simulink model "fuzzyLCSv2"  (R2021b)
settings: Solver=VariableStepAuto  StartTime=0.0  StopTime=inf  RelTol=1e-3
libraries: robotlib x3, fuzblock x1
settings Model: SimulationMode=accelerator  Creator=lucas  LastModifiedBy=lucas

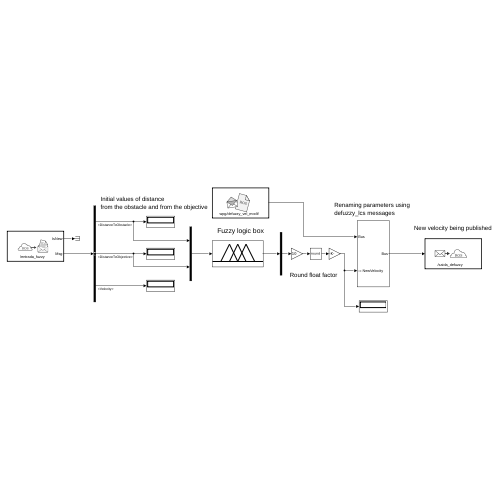
[thumbnail: Simulink's stored preview of the top-level diagram]
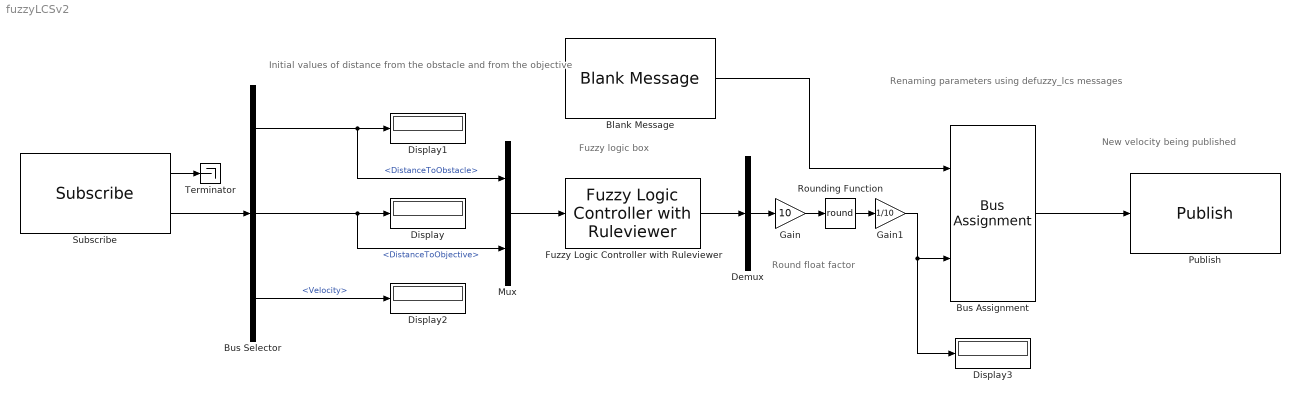
== system fuzzyLCSv2 ==
  note: Renaming parameters using
      | defuzzy_lcs messages
  note: Initial values of distance
      | from the obstacle and from the objective
  note: Fuzzy logic box
  note: New velocity being published
  note: Round float factor
  Blank Message : robotlib/Blank Message  messageClass=Message  entityType=wpg/defuzzy_vel_modif  messageType=wpg/defuzzy_vel_modif  SampleTime=inf  legacyBusStruct=off
  Bus Assignment : BusAssignment  AssignedSignals=NewVelocity
  Bus Selector : BusSelector  OutputSignals=DistanceToObstacle,DistanceToObjective,Velocity
  Demux : Demux  Outputs=1
  Display{,1..3} (4 alike) : Display
      settings: Decimation=2
  Fuzzy Logic Controller with Ruleviewer : fuzblock/Fuzzy Logic  Controller  with Ruleviewer  fismatrix=lucasdist  Ts=2
  Gain : Gain  Gain=10
  Gain1 : Gain  Gain=1/10
  Mux : Mux  Inputs=2
  Publish : robotlib/Publish  topicSource=Specify your own  topic=/saida_defuzzy  messageType=wpg/defuzzy_vel_modif  legacyBusStruct=off  messageQueueLength=1
  Rounding Function : Rounding  Operator=round
  Subscribe : robotlib/Subscribe  topicSource=Specify your own  topic=/entrada_fuzzy  messageType=wpg/fuzzy_vel_modif  SampleTime=-1  legacyBusStruct=off  messageQueueLength=1
  Terminator : Terminator
  wires:
  Subscribe/2 -> Bus Selector/1
  Subscribe/1 -> Terminator/1
  Bus Selector/1 -> Display1/1, Mux/1  "<DistanceToObstacle>"
  Bus Selector/2 -> Display/1, Mux/2  "<DistanceToObjective>"
  Bus Selector/3 -> Display2/1  "<Velocity>"
  Blank Message/1 -> Bus Assignment/1
  Bus Assignment/1 -> Publish/1
  Mux/1 -> Fuzzy Logic Controller with Ruleviewer/1
  Gain/1 -> Rounding Function/1
  Fuzzy Logic Controller with Ruleviewer/1 -> Demux/1
  Demux/1 -> Gain/1
  Rounding Function/1 -> Gain1/1
  Gain1/1 -> Display3/1, Bus Assignment/2
